simulink model "sim_001"  (R2021b)
settings: Solver=VariableStepAuto  StartTime=0.0  StopTime=10  RelTol=1e-3
values from neighbouring files (symbols this model uses):
  u_eq = z(4:5)    [f_003.m]
  x_eq = z(1:3)    [f_003.m]
undefined symbols (not defined in the file or in its folder): K
settings Model: Creator=Artun  LastModifiedBy=Artun

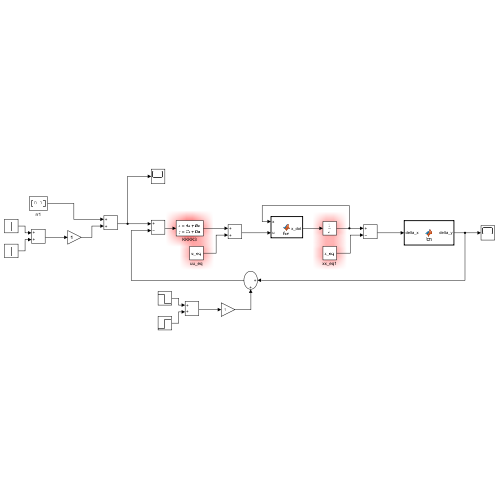
[thumbnail: Simulink's stored preview of the top-level diagram]
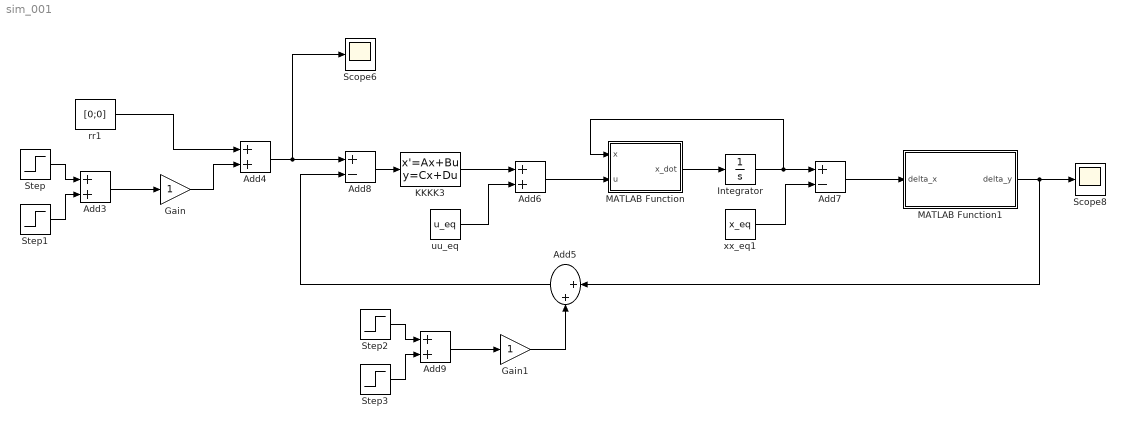
== system sim_001 ==
  Add{3..4,6,9} (4 alike) : Sum
  Add5 : Sum  Inputs=|++
  Add7 : Sum  Inputs=+-
  Add8 : Sum  Inputs=+-
  Gain : Gain
  Gain1 : Gain
  Integrator : Integrator  InitialCondition=x_eq
  KKKK3 : StateSpace  A=K.a  B=K.b  C=K.c  D=K.d  InitialCondition=0
  MATLAB Function : MATLAB Function  TreatAsAtomicUnit=on
  MATLAB Function1 : MATLAB Function  TreatAsAtomicUnit=on
  Scope6 : Scope
  Scope8 : Scope
  Step : Step  Time=1.1  After=-1  SampleTime=0
  Step1 : Step  SampleTime=0
  Step2 : Step  Time=5.1  After=-1  SampleTime=0
  Step3 : Step  Time=5  SampleTime=0
  rr1 : Constant  Value=[0;0]
  uu_eq : Constant  Value=u_eq
  xx_eq1 : Constant  Value=x_eq
  wires:
  rr1/1 -> Add4/1
  Step1/1 -> Add3/2
  Step/1 -> Add3/1
  Add3/1 -> Gain/1
  KKKK3/1 -> Add6/1
  uu_eq/1 -> Add6/2
  MATLAB Function/1(x_dot) -> Integrator/1
  Integrator/1 -> MATLAB Function/1(x), Add7/1
  xx_eq1/1 -> Add7/2
  Add7/1 -> MATLAB Function1/1(delta_x)
  Add6/1 -> MATLAB Function/2(u)
  Add4/1 -> Scope6/1, Add8/1
  MATLAB Function1/1(delta_y) -> Add5/1, Scope8/1
  Add8/1 -> KKKK3/1
  Gain/1 -> Add4/2
  Add5/1 -> Add8/2
  Add9/1 -> Gain1/1
  Step2/1 -> Add9/1
  Step3/1 -> Add9/2
  Gain1/1 -> Add5/2

== matlab function sim_001/MATLAB Function ==
  data: x input; u input; x_dot output
function x_dot = fcn(x, u)

u1=u(1);
u2=u(2);
x_dot=zeros(3,1);

A1=[5,-4,3;-5,5,3;-1,-5,4];
Q1=[-5,3,-3;-1,-1,-3;-3,5,-4];
Q2=[-4,1,1;4,-4,-2;1,4,0];
Q3=[-1,-4,-1;-5,-3,-5;-3,-3,4];

x_dot=A1*x+[x'*Q1*x;x'*Q2*x;x'*Q3*x]+[10;15;25]+[0;1;0]*u1+[0;0;1]*u2;

== matlab function sim_001/MATLAB Function1 ==
  data: delta_x input; delta_y output
function delta_y = fcn(delta_x)
delta_y=[1,0,0;0,1,0]*delta_x;
